simulink model "Control_Pendulo_Simple"  (R2021a)
settings: Solver=ode4  StartTime=0.0  StopTime=100  FixedStep=1e-3  RelTol=1e-3
PreLoadFcn:
  | Control_Pendulo_Simple_Cuentas;
InitFcn:
  | Control_Pendulo_Simple_Cuentas;
values from neighbouring files (symbols this model uses):
  K = acker(sys.A, sys.B, [-3 -3 -2 -2])    [Control_Pendulo_Simple_Cuentas.m]
  Ka = Ka(1:4)    [Control_Pendulo_Simple_Cuentas.m]
  KaDisc = KDisc2(1:4)    [Control_Pendulo_Simple_Cuentas.m]
  Kai = Ka(5)    [Control_Pendulo_Simple_Cuentas.m]
  KaiDisc = KDisc2(5)    [Control_Pendulo_Simple_Cuentas.m]
  KDisc = acker(sysDisc.A, sysDisc.B, exp([-2 -2 -1 -1].*Ts))    [Control_Pendulo_Simple_Cuentas.m]
  L = place((sys.A)',(sys.C)', [-25 -20 -35 -30])'    [Control_Pendulo_Simple_Cuentas.m]
  LDisc = place((sysDisc.A)',(sysDisc.C)', exp([-20 -15 -25 -30].*Ts))'    [Control_Pendulo_Simple_Cuentas.m]
  s = tf('s')    [Control_Pendulo_Simple_Cuentas.m]
  sys = ss(A,B,C,D)    [Control_Pendulo_Simple_Cuentas.m]
  sysDisc = c2d(sys, Ts, 'tustin')    [Control_Pendulo_Simple_Cuentas.m]
  Ts = 0.1    [Control_Pendulo_Simple_Cuentas.m]
  Ts2 = 0.05    [Control_Pendulo_Simple_Cuentas.m]
  Ts_loop = 25/1000    (= 0.025)    [Control_Pendulo_Simple_Cuentas.m]
undefined symbols (not defined in the file or in its folder): C_p_d, C_p_Disc_d, C_p_Disc_n, C_p_n, C_q_d, C_q_Disc_d, C_q_Disc_n, C_q_n, DiscIntNeverNeededParam, X, Y, Z
libraries: sm_lib x84, nesl_utility x42, eeGeneralControl x5
(part 1 of 3)
settings Model: Creator=Acer  LastModifiedBy=Acer

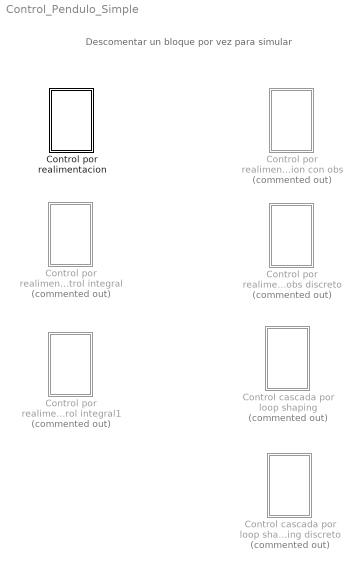
== system Control_Pendulo_Simple ==
  note: Descomentar un bloque por vez para simular
  Control cascada por loop shaping : Subsystem  Commented=on
  Control cascada por loop shaping discreto : Subsystem  Commented=on
  Control por realimentacion : Subsystem
  Control por realimentacion con control integral : Subsystem  Commented=on
  Control por realimentacion con control integral1 : Subsystem  Commented=on
  Control por realimentacion con obs : Subsystem  Commented=on
  Control por realimentacion con obs discreto : Subsystem  Commented=on

== system Control_Pendulo_Simple/Control cascada por loop shaping ==
  note: 2 seg -> Referencia de posición a 5m
      |
      | Notar el error permanente.
  note: Loop shaping de la posición
  Gain : Gain  Gain=-1
  Loop shaping del ángulo : Subsystem
  Pos y Ang : Scope  NumInputPorts=2
  Ref y Pos : Scope  NumInputPorts=2
  Step : Step  Time=2  SampleTime=0
  Sum : Sum  Inputs=|+-
  Transfer Fcn : TransferFcn  Numerator=C_p_n  Denominator=C_p_d
  wires:
  Sum/1 -> Loop shaping del ángulo/1(In1)
  Loop shaping del ángulo/1(Posicion) -> Transfer Fcn/1, Pos y Ang/1, Gain/1
  Loop shaping del ángulo/2(Angulo) -> Pos y Ang/2
  Transfer Fcn/1 -> Sum/2
  Step/1 -> Ref y Pos/1, Sum/1
  Gain/1 -> Ref y Pos/2

== system Control_Pendulo_Simple/Control cascada por loop shaping discreto ==
  note: 2 seg -> Referencia de posición a 5m
      |
      | Notar el error permanente.
  note: Loop shaping de la posición
  Discrete Transfer Fcn : DiscreteTransferFcn  Numerator=C_p_Disc_n  Denominator=C_p_Disc_d  SampleTime=Ts_loop
  Gain : Gain  Gain=-1
  Loop shaping del ángulo : Subsystem
  Pos y Ang : Scope  NumInputPorts=2
  Ref y Pos : Scope  NumInputPorts=2
  Step : Step  Time=2  SampleTime=0
  Sum : Sum  Inputs=|+-
  wires:
  Sum/1 -> Loop shaping del ángulo/1(In1)
  Loop shaping del ángulo/1(Posicion) -> Discrete Transfer Fcn/1, Pos y Ang/1, Gain/1
  Loop shaping del ángulo/2(Angulo) -> Pos y Ang/2
  Discrete Transfer Fcn/1 -> Sum/2
  Step/1 -> Ref y Pos/1, Sum/1
  Gain/1 -> Ref y Pos/2

== system Control_Pendulo_Simple/Control por realimentacion ==
  note: Control por realimentación:
      | 1 seg -> ref de posición a 5m
      | 12 seg -> ref de posición a -5m
      | 25 seg -> disturbio cada 3 segundos
      |
      | Notar el error permanente
  Disturbio : Subsystem
  Gain : Gain  Gain=-K  Multiplication=Matrix(K*u) (u vector)
  Gain1 : Gain  Gain=-1
  Mux : Mux
  Planta : Subsystem  mask{carro_masa=1, barra1_masa=0.25, barra1_long=8}
      mask prompts: carro_masa "Masa del carro"; barra1_masa "Masa primera barra"; barra1_long "Longitud primera barra"
  Pos y Ang : Scope  NumInputPorts=2
  Pos y Ref : Scope  NumInputPorts=2
  Referencia : Subsystem
  Sum : Sum  Inputs=|++
  Sum1 : Sum  Inputs=|++
  wires:
  Mux/1 -> Gain/1
  Planta/1(q) -> Mux/3, Pos y Ang/2  "Angulo"
  Planta/4(v) -> Mux/2  "Velocidad"
  Planta/2(w) -> Mux/4  "Vel Angular"
  Sum/1 -> Planta/1(u)
  Gain/1 -> Sum/2
  Planta/3(p) -> Pos y Ang/1, Pos y Ref/1, Sum1/2  "Posicion"
  Sum1/1 -> Mux/1
  Referencia/1(Posición) -> Gain1/1, Sum1/1
  Disturbio/1(F) -> Sum/1
  Gain1/1 -> Pos y Ref/2

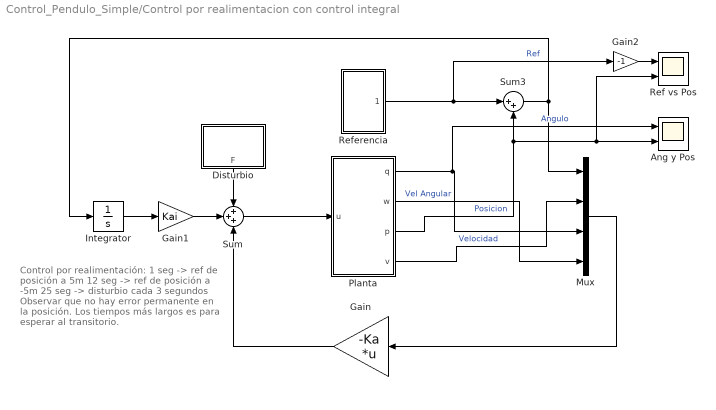
== system Control_Pendulo_Simple/Control por realimentacion con control integral ==
  note: Control por realimentación:
      | 1 seg -> ref de posición a 5m
      | 12 seg -> ref de posición a -5m
      | 25 seg -> disturbio cada 3 segundos
      |
      | Observar que no hay error permanente en la posición. Los tiempos más largos es para esperar al transitorio.
  Ang y Pos : Scope  NumInputPorts=2
  Disturbio : Subsystem
  Gain : Gain  Gain=-Ka  Multiplication=Matrix(K*u) (u vector)
  Gain1 : Gain  Gain=Kai
  Gain2 : Gain  Gain=-1
  Integrator : Integrator
  Mux : Mux
  Planta : Subsystem  mask{carro_masa=1, barra1_masa=0.25, barra1_long=8}
      mask prompts: carro_masa "Masa del carro"; barra1_masa "Masa primera barra"; barra1_long "Longitud primera barra"
  Ref vs Pos : Scope  NumInputPorts=2
  Referencia : Subsystem
  Sum : Sum  Inputs=+++
  Sum3 : Sum  Inputs=|++
  wires:
  Planta/1(q) -> Ang y Pos/1, Mux/3  "Angulo"
  Planta/4(v) -> Mux/2  "Velocidad"
  Gain1/1 -> Sum/2
  Planta/2(w) -> Mux/4  "Vel Angular"
  Sum/1 -> Planta/1(u)
  Mux/1 -> Gain/1
  Gain/1 -> Sum/3
  Sum3/1 -> Integrator/1, Mux/1
  Integrator/1 -> Gain1/1
  Planta/3(p) -> Sum3/2, Ref vs Pos/2, Ang y Pos/2  "Posicion"
  Referencia/1(Posición) -> Gain2/1, Sum3/1  "Ref"
  Disturbio/1(F) -> Sum/1
  Gain2/1 -> Ref vs Pos/1

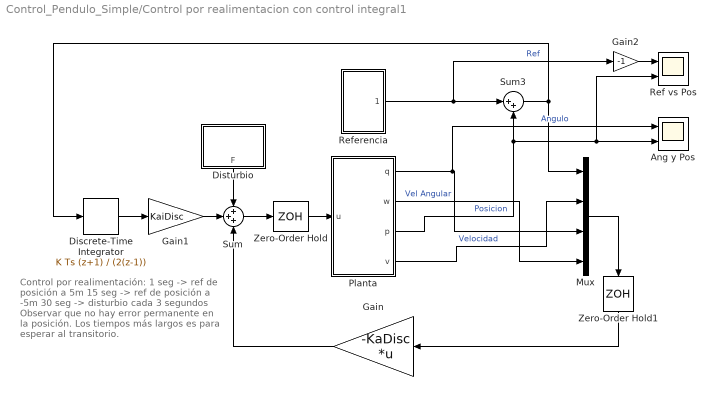
== system Control_Pendulo_Simple/Control por realimentacion con control integral1 ==
  note: Control por realimentación:
      | 1 seg -> ref de posición a 5m
      | 15 seg -> ref de posición a -5m
      | 30 seg -> disturbio cada 3 segundos
      |
      | Observar que no hay error permanente en la posición. Los tiempos más largos es para esperar al transitorio.
  Ang y Pos : Scope  NumInputPorts=2
  Discrete-Time Integrator : DiscreteIntegrator  IntegratorMethod=Integration: Trapezoidal  SampleTime=Ts2  ICPrevOutput=DiscIntNeverNeededParam  ICPrevScaledInput=DiscIntNeverNeededParam
  Disturbio : Subsystem
  Gain : Gain  Gain=-KaDisc  Multiplication=Matrix(K*u) (u vector)
  Gain1 : Gain  Gain=KaiDisc
  Gain2 : Gain  Gain=-1
  Mux : Mux
  Planta : Subsystem  mask{carro_masa=1, barra1_masa=0.25, barra1_long=8}
      mask prompts: carro_masa "Masa del carro"; barra1_masa "Masa primera barra"; barra1_long "Longitud primera barra"
  Ref vs Pos : Scope  NumInputPorts=2
  Referencia : Subsystem
  Sum : Sum  Inputs=+++
  Sum3 : Sum  Inputs=|++
  Zero-Order Hold : ZeroOrderHold  SampleTime=Ts2
  Zero-Order Hold1 : ZeroOrderHold  SampleTime=Ts2
  wires:
  Planta/1(q) -> Ang y Pos/1, Mux/3  "Angulo"
  Planta/4(v) -> Mux/2  "Velocidad"
  Gain1/1 -> Sum/2
  Planta/2(w) -> Mux/4  "Vel Angular"
  Sum/1 -> Zero-Order Hold/1
  Mux/1 -> Zero-Order Hold1/1
  Gain/1 -> Sum/3
  Sum3/1 -> Discrete-Time Integrator/1, Mux/1
  Discrete-Time Integrator/1 -> Gain1/1
  Planta/3(p) -> Sum3/2, Ref vs Pos/2, Ang y Pos/2  "Posicion"
  Referencia/1(Posición) -> Gain2/1, Sum3/1  "Ref"
  Disturbio/1(F) -> Sum/1
  Gain2/1 -> Ref vs Pos/1
  Zero-Order Hold/1 -> Planta/1(u)
  Zero-Order Hold1/1 -> Gain/1

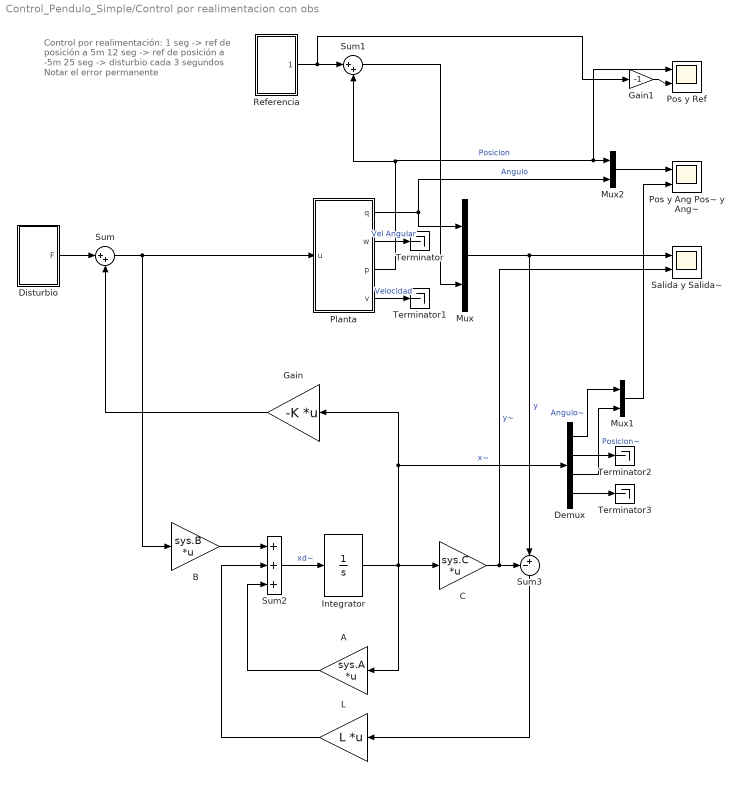
== system Control_Pendulo_Simple/Control por realimentacion con obs ==
  note: Control por realimentación:
      | 1 seg -> ref de posición a 5m
      | 12 seg -> ref de posición a -5m
      | 25 seg -> disturbio cada 3 segundos
      |
      | Notar el error permanente
  A : Gain  Gain=sys.A  Multiplication=Matrix(K*u) (u vector)
  B : Gain  Gain=sys.B  Multiplication=Matrix(K*u) (u vector)
  C : Gain  Gain=sys.C  Multiplication=Matrix(K*u) (u vector)
  Demux : Demux
  Disturbio : Subsystem
  Gain : Gain  Gain=-K  Multiplication=Matrix(K*u) (u vector)
  Gain1 : Gain  Gain=-1
  Integrator : Integrator  InitialCondition=[0 0 0 0]
  L : Gain  Gain=L  Multiplication=Matrix(K*u) (u vector)
  Mux : Mux  Inputs=2
  Mux1 : Mux  Inputs=2
  Mux2 : Mux  Inputs=2
  Planta : Subsystem  mask{carro_masa=1, barra1_masa=0.25, barra1_long=8}
      mask prompts: carro_masa "Masa del carro"; barra1_masa "Masa primera barra"; barra1_long "Longitud primera barra"
  Pos y Ang Pos~ y Ang~ : Scope  NumInputPorts=2
  Pos y Ref : Scope  NumInputPorts=2
  Referencia : Subsystem
  Salida y Salida~ : Scope  NumInputPorts=2
  Sum : Sum  Inputs=|++
  Sum1 : Sum  Inputs=|++
  Sum2 : Sum  Inputs=+++
  Sum3 : Sum  Inputs=-+|
  Terminator{,1..3} (4 alike) : Terminator
  wires:
  Sum/1 -> Planta/1(u), B/1
  Gain/1 -> Sum/2
  Disturbio/1(F) -> Sum/1
  Integrator/1 -> Demux/1, Gain/1, C/1, A/1  "x~"
  Sum2/1 -> Integrator/1  "xd~"
  A/1 -> Sum2/3
  B/1 -> Sum2/1
  Sum3/1 -> L/1
  L/1 -> Sum2/2
  C/1 -> Salida y Salida~/2, Sum3/1  "y~"
  Mux/1 -> Sum3/2, Salida y Salida~/1  "y"
  Sum1/1 -> Mux/2
  Referencia/1(Posición) -> Gain1/1, Sum1/1
  Gain1/1 -> Pos y Ref/2
  Planta/1(q) -> Mux2/2, Mux/1  "Angulo"
  Planta/3(p) -> Mux2/1, Pos y Ref/1, Sum1/2  "Posicion"
  Planta/2(w) -> Terminator/1  "Vel Angular"
  Planta/4(v) -> Terminator1/1  "Velocidad"
  Demux/1 -> Mux1/1  "Angulo~"
  Demux/3 -> Mux1/2  "Posicion~"
  Demux/2 -> Terminator2/1
  Demux/4 -> Terminator3/1
  Mux2/1 -> Pos y Ang Pos~ y Ang~/1
  Mux1/1 -> Pos y Ang Pos~ y Ang~/2

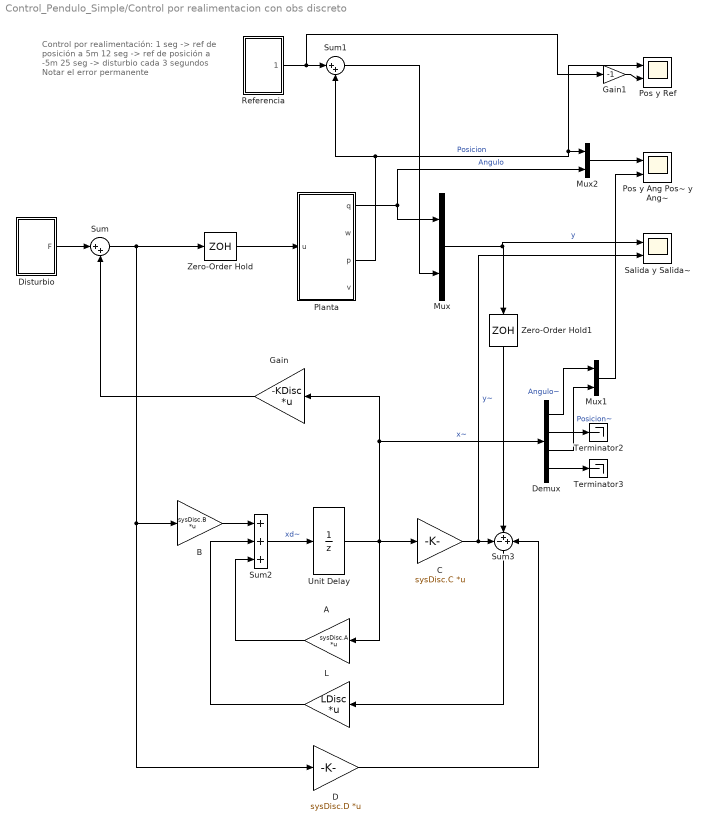
== system Control_Pendulo_Simple/Control por realimentacion con obs discreto ==
  note: Control por realimentación:
      | 1 seg -> ref de posición a 5m
      | 12 seg -> ref de posición a -5m
      | 25 seg -> disturbio cada 3 segundos
      |
      | Notar el error permanente
  A : Gain  Gain=sysDisc.A  Multiplication=Matrix(K*u) (u vector)
  B : Gain  Gain=sysDisc.B  Multiplication=Matrix(K*u) (u vector)
  C : Gain  Gain=sysDisc.C  Multiplication=Matrix(K*u) (u vector)
  D : Gain  Gain=sysDisc.D  Multiplication=Matrix(K*u) (u vector)
  Demux : Demux
  Disturbio : Subsystem
  Gain : Gain  Gain=-KDisc  Multiplication=Matrix(K*u) (u vector)
  Gain1 : Gain  Gain=-1
  L : Gain  Gain=LDisc  Multiplication=Matrix(K*u) (u vector)
  Mux : Mux  Inputs=2
  Mux1 : Mux  Inputs=2
  Mux2 : Mux  Inputs=2
  Planta : Subsystem  mask{carro_masa=1, barra1_masa=0.25, barra1_long=8}
      mask prompts: carro_masa "Masa del carro"; barra1_masa "Masa primera barra"; barra1_long "Longitud primera barra"
  Pos y Ang Pos~ y Ang~ : Scope  NumInputPorts=2
  Pos y Ref : Scope  NumInputPorts=2
  Referencia : Subsystem
  Salida y Salida~ : Scope  NumInputPorts=2
  Sum : Sum  Inputs=|++
  Sum1 : Sum  Inputs=|++
  Sum2 : Sum  Inputs=+++
  Sum3 : Sum  Inputs=-++
  Terminator2 : Terminator
  Terminator3 : Terminator
  Unit Delay : UnitDelay  InitialCondition=[0 0 0 0]  SampleTime=Ts  HasFrameUpgradeWarning=on
  Zero-Order Hold : ZeroOrderHold  SampleTime=Ts
  Zero-Order Hold1 : ZeroOrderHold  SampleTime=Ts
  wires:
  Sum/1 -> Zero-Order Hold/1, B/1, D/1
  Gain/1 -> Sum/2
  Disturbio/1(F) -> Sum/1
  Sum2/1 -> Unit Delay/1  "xd~"
  A/1 -> Sum2/3
  B/1 -> Sum2/1
  Sum3/1 -> L/1
  L/1 -> Sum2/2
  Sum1/1 -> Mux/2
  D/1 -> Sum3/3
  Zero-Order Hold/1 -> Planta/1(u)
  Zero-Order Hold1/1 -> Sum3/2
  Mux1/1 -> Pos y Ang Pos~ y Ang~/2
  Mux2/1 -> Pos y Ang Pos~ y Ang~/1
  Planta/3(p) -> Sum1/2, Mux2/1, Pos y Ref/1  "Posicion"
  Demux/2 -> Terminator2/1
  Demux/3 -> Mux1/2  "Posicion~"
  Planta/1(q) -> Mux2/2, Mux/1  "Angulo"
  Unit Delay/1 -> Demux/1, Gain/1, C/1, A/1  "x~"
  Referencia/1(Posición) -> Gain1/1, Sum1/1
  Mux/1 -> Salida y Salida~/1, Zero-Order Hold1/1  "y"
  Gain1/1 -> Pos y Ref/2
  Demux/1 -> Mux1/1  "Angulo~"
  C/1 -> Salida y Salida~/2, Sum3/1  "y~"
  Demux/4 -> Terminator3/1

== system Control_Pendulo_Simple/Control cascada por loop shaping/Loop shaping del ángulo ==
  In1 : Inport
  Planta : Subsystem  mask{carro_masa=1, barra1_masa=0.25, barra1_long=8}
      mask prompts: carro_masa "Masa del carro"; barra1_masa "Masa primera barra"; barra1_long "Longitud primera barra"
  Sum : Sum  Inputs=|+-
  Transfer Fcn : TransferFcn  Numerator=C_q_n  Denominator=C_q_d
  Posicion : Outport
  Angulo : Outport  Port=2
  wires:
  Planta/2(p) -> Posicion/1  "Posicion"
  Planta/1(q) -> Transfer Fcn/1, Angulo/1  "Angulo"
  In1/1 -> Sum/1
  Sum/1 -> Planta/1(u)
  Transfer Fcn/1 -> Sum/2

== system Control_Pendulo_Simple/Control cascada por loop shaping discreto/Loop shaping del ángulo ==
  In1 : Inport
  Discrete Transfer Fcn : DiscreteTransferFcn  Numerator=C_q_Disc_n  Denominator=C_q_Disc_d  SampleTime=Ts_loop
  Planta : Subsystem  mask{carro_masa=1, barra1_masa=0.25, barra1_long=8}
      mask prompts: carro_masa "Masa del carro"; barra1_masa "Masa primera barra"; barra1_long "Longitud primera barra"
  Sum : Sum  Inputs=|+-
  Zero-Order Hold : ZeroOrderHold  SampleTime=Ts_loop
  Zero-Order Hold1 : ZeroOrderHold  SampleTime=Ts_loop
  Zero-Order Hold2 : ZeroOrderHold  SampleTime=Ts_loop
  Posicion : Outport
  Angulo : Outport  Port=2
  wires:
  Planta/2(p) -> Zero-Order Hold2/1  "Posicion"
  Planta/1(q) -> Zero-Order Hold1/1  "Angulo"
  In1/1 -> Sum/1
  Sum/1 -> Zero-Order Hold/1
  Discrete Transfer Fcn/1 -> Sum/2
  Zero-Order Hold/1 -> Planta/1(u)
  Zero-Order Hold1/1 -> Discrete Transfer Fcn/1, Angulo/1
  Zero-Order Hold2/1 -> Posicion/1

== system Control_Pendulo_Simple/Control por realimentacion/Disturbio ==
  Pulse Generator : DiscretePulseGenerator  PulseType=Time based  Amplitude=500  Period=3  PulseWidth=0.5  PhaseDelay=25
  F : Outport
  wires:
  Pulse Generator/1 -> F/1

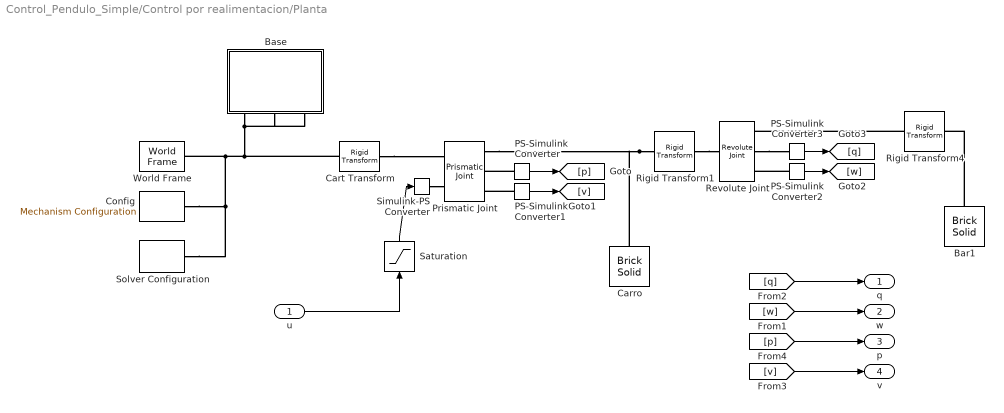
== system Control_Pendulo_Simple/Control por realimentacion/Planta ==
  u : Inport
  Bar1 : sm_lib/Body Elements/Brick Solid  GraphicAmbientColor=[0.15 0.15 0.15 1.0]  BasedOnType=Mass  BrickDimensions=[barra1_long 0.5 0.5]  BrickDimensionUnits=m  CenterOfMass=[0 0 0]  CenterOfMassUnits=m  GraphicDiffuseColor=[1.0 0 0]  Density=1000  DensityUnits=kg/m^3  DoExposeReferenceFrame=off  GraphicEmissiveColor=[0.0 0.0 0.0 1.0]  ExportEntireGeometry=off  SerializedFrames=<Frames><Frame><Id>Frame1</Id><Value><Name>F1</Name><Origin><Source>GeometricFeature</Source><FeatureName>+x surface</FeatureName></Origin><PrimaryAxis><DefinedDirection>+Z</DefinedDirection><Source>ReferenceFrame</Source><SourceDirection>+Z</SourceDirection><FeatureName></FeatureName></PrimaryAxis><SecondaryAxis><DefinedDirection>+X</DefinedDirection><Source>ReferenceFrame</Source><SourceDirection>+X</SourceDirection><FeatureName></FeatureName></SecondaryAxis></Value></Frame></Frames>  MarkerShape=Sphere  MarkerSize=10  GraphicType=FromGeometry  InertiaType=CalculateFromGeometry  Mass=barra1_masa  MassUnits=kg  MomentsOfInertia=[1 1 1]  MomentsOfInertiaUnits=kg*m^2  GraphicOpacity=1.0  ProductsOfInertia=[0 0 0]  ProductsOfInertiaUnits=kg*m^2  GraphicShininess=75  GraphicSpecularColor=[0.5 0.5 0.5 1.0]  GraphicVisPropType=SimpleVisualProperties
  Base : Subsystem
      settings: PortSchema="{\"entries\":[{\"content\":{\"sides\":[{\"content\":{\"connectorIds\":[]},\"type\":\"ConnectorPlacement.EquallySpacedRectSide\",\"uuid\":\"4332d69e-9bfe-4e89-a576-e2f6915cd745\"},{\"content\":{\"connectorIds\":[],\"side\":\"RIGHT\"},\"type\":\"ConnectorPlacement.EquallySpacedRectSide\",\"uuid\":\"1cc8b419-5de1-497b-b007-7cad9f99b098\"},{\"content\":{\"connectorIds\":[],\"side\":\"TOP\"},\"type\":\"ConnectorPlacement.EquallySpacedRectSide\",\"uuid\":\"21186588-641c-464a-a5f8-9ec189ea03bb\"},{\"content\":{\"connectorIds\":[\"RConn1\",\"RConn2\",\"RConn3\"],\"side\":\"BOTTOM\"},\"type\":\"ConnectorPlacement.EquallySpacedRectSide\",\"uuid\":\"3296c54c-d68e-452d-9e4e-a58ba512af2d\"}]},\"type\":\"ConnectorPlacement.EquallySpacedConnector\",\"uuid\":\"cf495630-4c35-4c65-b481-9d90798c8966\"}],\"packageUris\":[\"http://schema.mathworks.com/mf0/Connector/R2020b\"],\"version\":\"1.0\"}"
  Carro : sm_lib/Body Elements/Brick Solid  GraphicAmbientColor=[0.15 0.15 0.15 1.0]  BasedOnType=Mass  BrickDimensions=[0.5 1.5 3]  BrickDimensionUnits=m  CenterOfMass=[0 0 0]  CenterOfMassUnits=m  GraphicDiffuseColor=[1.0 1.0 1.0]  Density=1000  DensityUnits=kg/m^3  DoExposeReferenceFrame=on  GraphicEmissiveColor=[0.0 0.0 0.0 1.0]  ExportEntireGeometry=off  SerializedFrames=<Frames/>  MarkerShape=Sphere  MarkerSize=10  GraphicType=FromGeometry  InertiaType=CalculateFromGeometry  Mass=carro_masa  MassUnits=kg  MomentsOfInertia=[1 1 1]  MomentsOfInertiaUnits=kg*m^2  GraphicOpacity=1.0  ProductsOfInertia=[0 0 0]  ProductsOfInertiaUnits=kg*m^2  GraphicShininess=75  GraphicSpecularColor=[0.5 0.5 0.5 1.0]  GraphicVisPropType=SimpleVisualProperties
  Cart Transform : sm_lib/Frames and Transforms/Rigid Transform  TranslationMethod=StandardAxis  TranslationStandardOffset=0.2  TranslationLengthUnit=m  TranslationStandardAxis=+Z  TranslationCartesianOffset=[0 0 0]  TranslationROffset=0  TranslationROffsetUnits=m  TranslationZOffset=0  TranslationZOffsetUnits=m  TranslationThetaOffset=0  TranslationThetaOffsetUnits=deg  RotationMethod=RotationSequence  RotationAngleUnits=deg  RotationStandardAxis=+Z  RotationAngle=0.0  RotationArbitraryAxis=[0 0 1]  FollAlignAxisA=+X  BaseAlignAxisA=+Y  FollAlignAxisB=+Y  BaseAlignAxisB=+Z  RotationSequenceAxes=FollowerAxes  RotationSequence=XYZ  RotationSequenceAngles=[0 90 0]  RotationSequenceAnglesUnits=deg  RotationMatrix=[1 0 0; 0 1 0; 0 0 1]
  Config : sm_lib/Utilities/Mechanism Configuration  UniformGravity=Constant  GravityVector=[0 0 -9.81]  GravityVectorUnits=m/s^2  GravityUnits=m/s^2  LinearizationDelta=0.001  JointModeTransitionNonlinearIterations=2
  PS-Simulink Converter{,1..3} (4 alike) : nesl_utility/PS-Simulink Converter  PhysicalDomain=network_engine_domain  SubClassName=ps_output  LeftPortType=input  RightPortType=output  PseudoPeriodic=off  Frequencies=[]  Unit=inherit  AffineConversion=off
      settings: SourceProductBaseCode=PW,SS
  Prismatic Joint : sm_lib/Joints/Prismatic Joint  JointMode=Normal  SenseConstraintForce=off  SenseConstraintForceX=off  SenseConstraintForceY=off  SenseConstraintForceZ=off  SenseConstraintTorque=off  SenseConstraintTorqueX=off  SenseConstraintTorqueY=off  SenseConstraintTorqueZ=off  SenseTotalForce=off  SenseTotalForceX=off  SenseTotalForceY=off  SenseTotalForceZ=off  SenseTotalTorque=off  SenseTotalTorqueX=off  SenseTotalTorqueY=off  SenseTotalTorqueZ=off  CompositeWrenchDir=FollowerOnBase  CompositeWrenchFrame=BaseFrame  EquilibriumPosition=0  EquilibriumPositionUnits=m  SpringStiffness=0  SpringStiffnessUnits=N/m  DampingCoefficient=0  DampingCoefficientUnits=N/(m/s)  TorqueActuationMode=InputTorque  MotionActuationMode=ComputedMotion  SensePosition=on  SenseVelocity=on  SenseAcceleration=off  SenseTorqueForce=off  SenseLowerLimitTorqueForce=off  SenseUpperLimitTorqueForce=off  LowerLimitSpecify=off  LowerLimitBound=-10  LowerLimitBoundUnits=m  LowerLimitStiffness=1e6  LowerLimitStiffnessUnits=N/m  LowerLimitDamping=1e3  LowerLimitDampingUnits=N/(m/s)  LowerLimitTransitionRegionWidth=1e-4  LowerLimitTransitionRegionWidthUnits=m  UpperLimitSpecify=off  UpperLimitBound=10  UpperLimitBoundUnits=m  UpperLimitStiffness=1e6  UpperLimitStiffnessUnits=N/m  UpperLimitDamping=1e3  UpperLimitDampingUnits=N/(m/s)  UpperLimitTransitionRegionWidth=1e-4  UpperLimitTransitionRegionWidthUnits=m  PositionTargetSpecify=off  PositionTargetPriority=High  PositionTargetValue=0  PositionTargetValueUnits=m  VelocityTargetSpecify=off  VelocityTargetPriority=High  VelocityTargetValue=0  VelocityTargetValueUnits=m/s
  Revolute Joint : sm_lib/Joints/Revolute Joint  JointMode=Normal  SenseConstraintForce=off  SenseConstraintForceX=off  SenseConstraintForceY=off  SenseConstraintForceZ=off  SenseConstraintTorque=off  SenseConstraintTorqueX=off  SenseConstraintTorqueY=off  SenseConstraintTorqueZ=off  SenseTotalForce=off  SenseTotalForceX=off  SenseTotalForceY=off  SenseTotalForceZ=off  SenseTotalTorque=off  SenseTotalTorqueX=off  SenseTotalTorqueY=off  SenseTotalTorqueZ=off  CompositeWrenchDir=FollowerOnBase  CompositeWrenchFrame=BaseFrame  EquilibriumPosition=0  EquilibriumPositionUnits=deg  SpringStiffness=0  SpringStiffnessUnits=N*m/deg  DampingCoefficient=0  DampingCoefficientUnits=N*m/(deg/s)  TorqueActuationMode=NoTorque  MotionActuationMode=ComputedMotion  SensePosition=on  SenseVelocity=on  SenseAcceleration=off  SenseTorqueForce=off  SenseLowerLimitTorqueForce=off  SenseUpperLimitTorqueForce=off  LowerLimitSpecify=off  LowerLimitBound=-90  LowerLimitBoundUnits=deg  LowerLimitStiffness=1e4  LowerLimitStiffnessUnits=N*m/deg  LowerLimitDamping=10  LowerLimitDampingUnits=N*m/(deg/s)  LowerLimitTransitionRegionWidth=0.1  LowerLimitTransitionRegionWidthUnits=deg  UpperLimitSpecify=off  UpperLimitBound=90  UpperLimitBoundUnits=deg  UpperLimitStiffness=1e4  UpperLimitStiffnessUnits=N*m/deg  UpperLimitDamping=10  UpperLimitDampingUnits=N*m/(deg/s)  UpperLimitTransitionRegionWidth=0.1  UpperLimitTransitionRegionWidthUnits=deg  PositionTargetSpecify=off  PositionTargetPriority=Low  PositionTargetValue=0.001  PositionTargetValueUnits=deg  VelocityTargetSpecify=off  VelocityTargetPriority=High  VelocityTargetValue=0  VelocityTargetValueUnits=deg/s
  Rigid Transform1 : sm_lib/Frames and Transforms/Rigid Transform  TranslationMethod=StandardAxis  TranslationStandardOffset=0  TranslationLengthUnit=m  TranslationStandardAxis=+X  TranslationCartesianOffset=[0 0 0]  TranslationROffset=0  TranslationROffsetUnits=m  TranslationZOffset=0  TranslationZOffsetUnits=m  TranslationThetaOffset=0  TranslationThetaOffsetUnits=deg  RotationMethod=RotationSequence  RotationAngleUnits=deg  RotationStandardAxis=+Z  RotationAngle=0.0  RotationArbitraryAxis=[0 0 1]  FollAlignAxisA=+X  BaseAlignAxisA=+Y  FollAlignAxisB=+Y  BaseAlignAxisB=+Z  RotationSequenceAxes=FollowerAxes  RotationSequence=XYZ  RotationSequenceAngles=[90 0 0.1]  RotationSequenceAnglesUnits=deg  RotationMatrix=[1 0 0; 0 1 0; 0 0 1]
  Rigid Transform4 : sm_lib/Frames and Transforms/Rigid Transform  TranslationMethod=StandardAxis  TranslationStandardOffset=0  TranslationLengthUnit=m  TranslationStandardAxis=+Z  TranslationCartesianOffset=[0 0 0]  TranslationROffset=0  TranslationROffsetUnits=m  TranslationZOffset=0  TranslationZOffsetUnits=m  TranslationThetaOffset=0  TranslationThetaOffsetUnits=deg  RotationMethod=RotationSequence  RotationAngleUnits=deg  RotationStandardAxis=+Z  RotationAngle=0.0  RotationArbitraryAxis=[0 0 1]  FollAlignAxisA=+X  BaseAlignAxisA=+Y  FollAlignAxisB=+Y  BaseAlignAxisB=+Z  RotationSequenceAxes=FollowerAxes  RotationSequence=XYZ  RotationSequenceAngles=[0 0 0]  RotationSequenceAnglesUnits=deg  RotationMatrix=[1 0 0; 0 1 0; 0 0 1]
  Saturation : Saturate  UpperLimit=1000  LowerLimit=-1000
  Simulink-PS Converter : nesl_utility/Simulink-PS Converter  PhysicalDomain=network_engine_domain  SubClassName=ps_input  LeftPortType=input  RightPortType=output  PseudoPeriodic=off  Frequencies=[]  NoiseDistribution=none  NoiseParameters=[]  Unit=1  AffineConversion=off  FilteringAndDerivatives=provide  SimscapeFilterOrder=1  InputFilterTimeConstant=0.001  UdotUserProvided=0
      settings: SourceProductBaseCode=PW,SS
  Solver Configuration : nesl_utility/Solver Configuration  PhysicalDomain=network_engine_domain  SubClassName=solver  LeftPortType=input  RightPortType=generic  Tones=[]  Harmonics=[]  SimulateNoise=off  Profile=off  UseLocalSampling=off  EnableSwitchedLinearOptims=on  FrequencyDomain=off  UseCCode=off  RelTol=0.001  AbsTol=1e-06  MinStep=1e-09  ToWorkspace=off  RevertToSquareIcSolve=off  NumHomotopyIterations=100  PhasorMode=off  PhasorModeNumHarmonics=1  DoDC=off  ResidualTolerance=1e-09  UseLocalSolver=off  LocalSolverChoice=NE_BACKWARD_EULER_ADVANCER  LocalSolverSampleTime=0.001  DoFixedCost=off  MaxNonlinIter=3  MaxModeIter=2  ComputeImpulses=off  ImpulseIterations=2  LinearAlgebra=auto  EquationFormulation=NE_TIME_EF  DelaysMemoryBudget=1024  AutomaticFiltering=on  FilteringTimeConstant=0.001  PartitionStorageMethod=AS_NEEDED  PartitionMemoryBudget=1024  PartitionMethod=ROBUST
      settings: SourceProductBaseCode=PW,SS
  World Frame : sm_lib/Frames and Transforms/World Frame
  q : Outport
  w : Outport  Port=2
  p : Outport  Port=3
  v : Outport  Port=4
  wires:
  u/1 -> Saturation/1
  PS-Simulink Converter/1 -> [p]
  PS-Simulink Converter3/1 -> [q]
  [q] -> q/1
  [p] -> p/1
  PS-Simulink Converter1/1 -> [v]
  PS-Simulink Converter2/1 -> [w]
  [w] -> w/1
  [v] -> v/1
  Saturation/1 -> Simulink-PS Converter/1
  connections:
  PS-Simulink Converter1/LConn1 -- Prismatic Joint/RConn3
  Bar1/LConn1 -- Rigid Transform4/RConn1
  Rigid Transform4/LConn1 -- Revolute Joint/RConn1
  Config/RConn1 -- Solver Configuration/RConn1 -- Cart Transform/LConn1 -- Base/RConn3 -- Base/RConn2 -- Base/RConn1 -- World Frame/RConn1
  Cart Transform/RConn1 -- Prismatic Joint/LConn1
  PS-Simulink Converter/LConn1 -- Prismatic Joint/RConn2
  Simulink-PS Converter/RConn1 -- Prismatic Joint/LConn2
  PS-Simulink Converter2/LConn1 -- Revolute Joint/RConn3
  Rigid Transform1/RConn1 -- Revolute Joint/LConn1
  Revolute Joint/RConn2 -- PS-Simulink Converter3/LConn1
  Rigid Transform1/LConn1 -- Prismatic Joint/RConn1 -- Carro/RConn1

== system Control_Pendulo_Simple/Control por realimentacion/Referencia ==
  note: Pre-filtro para no irse mucho del punto de linealización
  Low-Pass Filter (Discrete or Continuous) : eeGeneralControl/Low-Pass Filter (Discrete or Continuous)  K=1  T=1  B=inf  A=-inf  init_option=Inherited from block input  x0=0  Ts=-1
  Step1 : Step  After=2  SampleTime=0
  Step2 : Step  Time=12  After=-4  SampleTime=0
  Sum2 : Sum  Inputs=|++
  Posición : Outport
  wires:
  Step2/1 -> Sum2/2
  Sum2/1 -> Low-Pass Filter (Discrete or Continuous)/1
  Low-Pass Filter (Discrete or Continuous)/1 -> Posición/1
  Step1/1 -> Sum2/1

== system Control_Pendulo_Simple/Control por realimentacion con control integral/Disturbio ==
  Pulse Generator : DiscretePulseGenerator  PulseType=Time based  Amplitude=500  Period=5  PulseWidth=0.5  PhaseDelay=25
  F : Outport
  wires:
  Pulse Generator/1 -> F/1

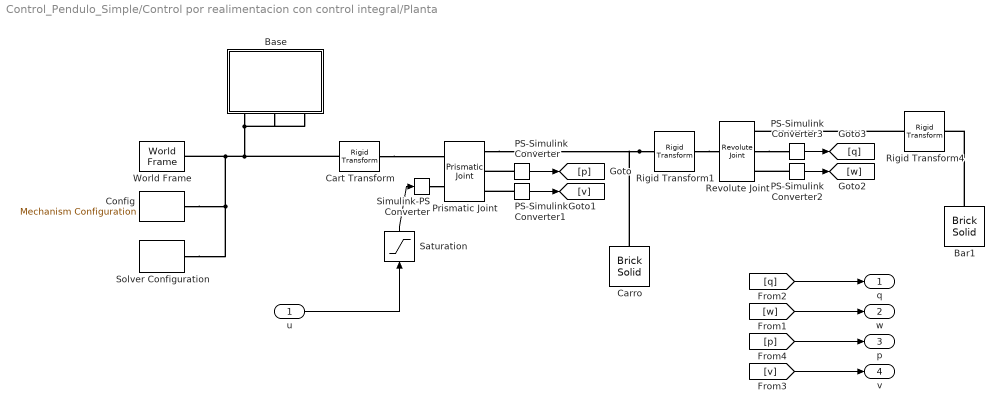
== system Control_Pendulo_Simple/Control por realimentacion con control integral/Planta ==
  u : Inport
  Bar1 : sm_lib/Body Elements/Brick Solid  GraphicAmbientColor=[0.15 0.15 0.15 1.0]  BasedOnType=Mass  BrickDimensions=[barra1_long 0.5 0.5]  BrickDimensionUnits=m  CenterOfMass=[0 0 0]  CenterOfMassUnits=m  GraphicDiffuseColor=[1.0 0 0]  Density=1000  DensityUnits=kg/m^3  DoExposeReferenceFrame=off  GraphicEmissiveColor=[0.0 0.0 0.0 1.0]  ExportEntireGeometry=off  SerializedFrames=<Frames><Frame><Id>Frame1</Id><Value><Name>F1</Name><Origin><Source>GeometricFeature</Source><FeatureName>+x surface</FeatureName></Origin><PrimaryAxis><DefinedDirection>+Z</DefinedDirection><Source>ReferenceFrame</Source><SourceDirection>+Z</SourceDirection><FeatureName></FeatureName></PrimaryAxis><SecondaryAxis><DefinedDirection>+X</DefinedDirection><Source>ReferenceFrame</Source><SourceDirection>+X</SourceDirection><FeatureName></FeatureName></SecondaryAxis></Value></Frame></Frames>  MarkerShape=Sphere  MarkerSize=10  GraphicType=FromGeometry  InertiaType=CalculateFromGeometry  Mass=barra1_masa  MassUnits=kg  MomentsOfInertia=[1 1 1]  MomentsOfInertiaUnits=kg*m^2  GraphicOpacity=1.0  ProductsOfInertia=[0 0 0]  ProductsOfInertiaUnits=kg*m^2  GraphicShininess=75  GraphicSpecularColor=[0.5 0.5 0.5 1.0]  GraphicVisPropType=SimpleVisualProperties
  Base : Subsystem
      settings: PortSchema="{\"entries\":[{\"content\":{\"sides\":[{\"content\":{\"connectorIds\":[]},\"type\":\"ConnectorPlacement.EquallySpacedRectSide\",\"uuid\":\"4332d69e-9bfe-4e89-a576-e2f6915cd745\"},{\"content\":{\"connectorIds\":[],\"side\":\"RIGHT\"},\"type\":\"ConnectorPlacement.EquallySpacedRectSide\",\"uuid\":\"1cc8b419-5de1-497b-b007-7cad9f99b098\"},{\"content\":{\"connectorIds\":[],\"side\":\"TOP\"},\"type\":\"ConnectorPlacement.EquallySpacedRectSide\",\"uuid\":\"21186588-641c-464a-a5f8-9ec189ea03bb\"},{\"content\":{\"connectorIds\":[\"RConn1\",\"RConn2\",\"RConn3\"],\"side\":\"BOTTOM\"},\"type\":\"ConnectorPlacement.EquallySpacedRectSide\",\"uuid\":\"3296c54c-d68e-452d-9e4e-a58ba512af2d\"}]},\"type\":\"ConnectorPlacement.EquallySpacedConnector\",\"uuid\":\"cf495630-4c35-4c65-b481-9d90798c8966\"}],\"packageUris\":[\"http://schema.mathworks.com/mf0/Connector/R2020b\"],\"version\":\"1.0\"}"
  Carro : sm_lib/Body Elements/Brick Solid  GraphicAmbientColor=[0.15 0.15 0.15 1.0]  BasedOnType=Mass  BrickDimensions=[0.5 1.5 3]  BrickDimensionUnits=m  CenterOfMass=[0 0 0]  CenterOfMassUnits=m  GraphicDiffuseColor=[1.0 1.0 1.0]  Density=1000  DensityUnits=kg/m^3  DoExposeReferenceFrame=on  GraphicEmissiveColor=[0.0 0.0 0.0 1.0]  ExportEntireGeometry=off  SerializedFrames=<Frames/>  MarkerShape=Sphere  MarkerSize=10  GraphicType=FromGeometry  InertiaType=CalculateFromGeometry  Mass=carro_masa  MassUnits=kg  MomentsOfInertia=[1 1 1]  MomentsOfInertiaUnits=kg*m^2  GraphicOpacity=1.0  ProductsOfInertia=[0 0 0]  ProductsOfInertiaUnits=kg*m^2  GraphicShininess=75  GraphicSpecularColor=[0.5 0.5 0.5 1.0]  GraphicVisPropType=SimpleVisualProperties
  Cart Transform : sm_lib/Frames and Transforms/Rigid Transform  TranslationMethod=StandardAxis  TranslationStandardOffset=0.2  TranslationLengthUnit=m  TranslationStandardAxis=+Z  TranslationCartesianOffset=[0 0 0]  TranslationROffset=0  TranslationROffsetUnits=m  TranslationZOffset=0  TranslationZOffsetUnits=m  TranslationThetaOffset=0  TranslationThetaOffsetUnits=deg  RotationMethod=RotationSequence  RotationAngleUnits=deg  RotationStandardAxis=+Z  RotationAngle=0.0  RotationArbitraryAxis=[0 0 1]  FollAlignAxisA=+X  BaseAlignAxisA=+Y  FollAlignAxisB=+Y  BaseAlignAxisB=+Z  RotationSequenceAxes=FollowerAxes  RotationSequence=XYZ  RotationSequenceAngles=[0 90 0]  RotationSequenceAnglesUnits=deg  RotationMatrix=[1 0 0; 0 1 0; 0 0 1]
  Config : sm_lib/Utilities/Mechanism Configuration  UniformGravity=Constant  GravityVector=[0 0 -9.81]  GravityVectorUnits=m/s^2  GravityUnits=m/s^2  LinearizationDelta=0.001  JointModeTransitionNonlinearIterations=2
  PS-Simulink Converter{,1..3} (4 alike) : nesl_utility/PS-Simulink Converter  PhysicalDomain=network_engine_domain  SubClassName=ps_output  LeftPortType=input  RightPortType=output  PseudoPeriodic=off  Frequencies=[]  Unit=inherit  AffineConversion=off
      settings: SourceProductBaseCode=PW,SS
  Prismatic Joint : sm_lib/Joints/Prismatic Joint  JointMode=Normal  SenseConstraintForce=off  SenseConstraintForceX=off  SenseConstraintForceY=off  SenseConstraintForceZ=off  SenseConstraintTorque=off  SenseConstraintTorqueX=off  SenseConstraintTorqueY=off  SenseConstraintTorqueZ=off  SenseTotalForce=off  SenseTotalForceX=off  SenseTotalForceY=off  SenseTotalForceZ=off  SenseTotalTorque=off  SenseTotalTorqueX=off  SenseTotalTorqueY=off  SenseTotalTorqueZ=off  CompositeWrenchDir=FollowerOnBase  CompositeWrenchFrame=BaseFrame  EquilibriumPosition=0  EquilibriumPositionUnits=m  SpringStiffness=0  SpringStiffnessUnits=N/m  DampingCoefficient=0  DampingCoefficientUnits=N/(m/s)  TorqueActuationMode=InputTorque  MotionActuationMode=ComputedMotion  SensePosition=on  SenseVelocity=on  SenseAcceleration=off  SenseTorqueForce=off  SenseLowerLimitTorqueForce=off  SenseUpperLimitTorqueForce=off  LowerLimitSpecify=off  LowerLimitBound=-10  LowerLimitBoundUnits=m  LowerLimitStiffness=1e6  LowerLimitStiffnessUnits=N/m  LowerLimitDamping=1e3  LowerLimitDampingUnits=N/(m/s)  LowerLimitTransitionRegionWidth=1e-4  LowerLimitTransitionRegionWidthUnits=m  UpperLimitSpecify=off  UpperLimitBound=10  UpperLimitBoundUnits=m  UpperLimitStiffness=1e6  UpperLimitStiffnessUnits=N/m  UpperLimitDamping=1e3  UpperLimitDampingUnits=N/(m/s)  UpperLimitTransitionRegionWidth=1e-4  UpperLimitTransitionRegionWidthUnits=m  PositionTargetSpecify=off  PositionTargetPriority=High  PositionTargetValue=0  PositionTargetValueUnits=m  VelocityTargetSpecify=off  VelocityTargetPriority=High  VelocityTargetValue=0  VelocityTargetValueUnits=m/s
  Revolute Joint : sm_lib/Joints/Revolute Joint  JointMode=Normal  SenseConstraintForce=off  SenseConstraintForceX=off  SenseConstraintForceY=off  SenseConstraintForceZ=off  SenseConstraintTorque=off  SenseConstraintTorqueX=off  SenseConstraintTorqueY=off  SenseConstraintTorqueZ=off  SenseTotalForce=off  SenseTotalForceX=off  SenseTotalForceY=off  SenseTotalForceZ=off  SenseTotalTorque=off  SenseTotalTorqueX=off  SenseTotalTorqueY=off  SenseTotalTorqueZ=off  CompositeWrenchDir=FollowerOnBase  CompositeWrenchFrame=BaseFrame  EquilibriumPosition=0  EquilibriumPositionUnits=deg  SpringStiffness=0  SpringStiffnessUnits=N*m/deg  DampingCoefficient=0  DampingCoefficientUnits=N*m/(deg/s)  TorqueActuationMode=NoTorque  MotionActuationMode=ComputedMotion  SensePosition=on  SenseVelocity=on  SenseAcceleration=off  SenseTorqueForce=off  SenseLowerLimitTorqueForce=off  SenseUpperLimitTorqueForce=off  LowerLimitSpecify=off  LowerLimitBound=-90  LowerLimitBoundUnits=deg  LowerLimitStiffness=1e4  LowerLimitStiffnessUnits=N*m/deg  LowerLimitDamping=10  LowerLimitDampingUnits=N*m/(deg/s)  LowerLimitTransitionRegionWidth=0.1  LowerLimitTransitionRegionWidthUnits=deg  UpperLimitSpecify=off  UpperLimitBound=90  UpperLimitBoundUnits=deg  UpperLimitStiffness=1e4  UpperLimitStiffnessUnits=N*m/deg  UpperLimitDamping=10  UpperLimitDampingUnits=N*m/(deg/s)  UpperLimitTransitionRegionWidth=0.1  UpperLimitTransitionRegionWidthUnits=deg  PositionTargetSpecify=off  PositionTargetPriority=Low  PositionTargetValue=0.001  PositionTargetValueUnits=deg  VelocityTargetSpecify=off  VelocityTargetPriority=High  VelocityTargetValue=0  VelocityTargetValueUnits=deg/s
  Rigid Transform1 : sm_lib/Frames and Transforms/Rigid Transform  TranslationMethod=StandardAxis  TranslationStandardOffset=0  TranslationLengthUnit=m  TranslationStandardAxis=+X  TranslationCartesianOffset=[0 0 0]  TranslationROffset=0  TranslationROffsetUnits=m  TranslationZOffset=0  TranslationZOffsetUnits=m  TranslationThetaOffset=0  TranslationThetaOffsetUnits=deg  RotationMethod=RotationSequence  RotationAngleUnits=deg  RotationStandardAxis=+Z  RotationAngle=0.0  RotationArbitraryAxis=[0 0 1]  FollAlignAxisA=+X  BaseAlignAxisA=+Y  FollAlignAxisB=+Y  BaseAlignAxisB=+Z  RotationSequenceAxes=FollowerAxes  RotationSequence=XYZ  RotationSequenceAngles=[90 0 0.1]  RotationSequenceAnglesUnits=deg  RotationMatrix=[1 0 0; 0 1 0; 0 0 1]
  Rigid Transform4 : sm_lib/Frames and Transforms/Rigid Transform  TranslationMethod=StandardAxis  TranslationStandardOffset=0  TranslationLengthUnit=m  TranslationStandardAxis=+Z  TranslationCartesianOffset=[0 0 0]  TranslationROffset=0  TranslationROffsetUnits=m  TranslationZOffset=0  TranslationZOffsetUnits=m  TranslationThetaOffset=0  TranslationThetaOffsetUnits=deg  RotationMethod=RotationSequence  RotationAngleUnits=deg  RotationStandardAxis=+Z  RotationAngle=0.0  RotationArbitraryAxis=[0 0 1]  FollAlignAxisA=+X  BaseAlignAxisA=+Y  FollAlignAxisB=+Y  BaseAlignAxisB=+Z  RotationSequenceAxes=FollowerAxes  RotationSequence=XYZ  RotationSequenceAngles=[0 0 0]  RotationSequenceAnglesUnits=deg  RotationMatrix=[1 0 0; 0 1 0; 0 0 1]
  Saturation : Saturate  UpperLimit=1000  LowerLimit=-1000
  Simulink-PS Converter : nesl_utility/Simulink-PS Converter  PhysicalDomain=network_engine_domain  SubClassName=ps_input  LeftPortType=input  RightPortType=output  PseudoPeriodic=off  Frequencies=[]  NoiseDistribution=none  NoiseParameters=[]  Unit=1  AffineConversion=off  FilteringAndDerivatives=provide  SimscapeFilterOrder=1  InputFilterTimeConstant=0.001  UdotUserProvided=0
      settings: SourceProductBaseCode=PW,SS
  Solver Configuration : nesl_utility/Solver Configuration  PhysicalDomain=network_engine_domain  SubClassName=solver  LeftPortType=input  RightPortType=generic  Tones=[]  Harmonics=[]  SimulateNoise=off  Profile=off  UseLocalSampling=off  EnableSwitchedLinearOptims=on  FrequencyDomain=off  UseCCode=off  RelTol=0.001  AbsTol=1e-06  MinStep=1e-09  ToWorkspace=off  RevertToSquareIcSolve=off  NumHomotopyIterations=100  PhasorMode=off  PhasorModeNumHarmonics=1  DoDC=off  ResidualTolerance=1e-09  UseLocalSolver=off  LocalSolverChoice=NE_BACKWARD_EULER_ADVANCER  LocalSolverSampleTime=0.001  DoFixedCost=off  MaxNonlinIter=3  MaxModeIter=2  ComputeImpulses=off  ImpulseIterations=2  LinearAlgebra=auto  EquationFormulation=NE_TIME_EF  DelaysMemoryBudget=1024  AutomaticFiltering=on  FilteringTimeConstant=0.001  PartitionStorageMethod=AS_NEEDED  PartitionMemoryBudget=1024  PartitionMethod=ROBUST
      settings: SourceProductBaseCode=PW,SS
  World Frame : sm_lib/Frames and Transforms/World Frame
  q : Outport
  w : Outport  Port=2
  p : Outport  Port=3
  v : Outport  Port=4
  wires:
  u/1 -> Saturation/1
  PS-Simulink Converter/1 -> [p]
  PS-Simulink Converter3/1 -> [q]
  [q] -> q/1
  [p] -> p/1
  PS-Simulink Converter1/1 -> [v]
  PS-Simulink Converter2/1 -> [w]
  [w] -> w/1
  [v] -> v/1
  Saturation/1 -> Simulink-PS Converter/1
  connections:
  PS-Simulink Converter1/LConn1 -- Prismatic Joint/RConn3
  Bar1/LConn1 -- Rigid Transform4/RConn1
  Rigid Transform4/LConn1 -- Revolute Joint/RConn1
  Config/RConn1 -- Solver Configuration/RConn1 -- Cart Transform/LConn1 -- Base/RConn3 -- Base/RConn2 -- Base/RConn1 -- World Frame/RConn1
  Cart Transform/RConn1 -- Prismatic Joint/LConn1
  PS-Simulink Converter/LConn1 -- Prismatic Joint/RConn2
  Simulink-PS Converter/RConn1 -- Prismatic Joint/LConn2
  PS-Simulink Converter2/LConn1 -- Revolute Joint/RConn3
  Rigid Transform1/RConn1 -- Revolute Joint/LConn1
  Revolute Joint/RConn2 -- PS-Simulink Converter3/LConn1
  Rigid Transform1/LConn1 -- Prismatic Joint/RConn1 -- Carro/RConn1

== system Control_Pendulo_Simple/Control por realimentacion con control integral/Referencia ==
  note: Pre-filtro para no irse mucho del punto de linealización
  Low-Pass Filter (Discrete or Continuous) : eeGeneralControl/Low-Pass Filter (Discrete or Continuous)  K=1  T=1  B=inf  A=-inf  init_option=Inherited from block input  x0=0  Ts=-1
  Step1 : Step  After=2  SampleTime=0
  Step2 : Step  Time=12  After=-4  SampleTime=0
  Sum2 : Sum  Inputs=|++
  Posición : Outport
  wires:
  Step2/1 -> Sum2/2
  Sum2/1 -> Low-Pass Filter (Discrete or Continuous)/1
  Low-Pass Filter (Discrete or Continuous)/1 -> Posición/1
  Step1/1 -> Sum2/1

== system Control_Pendulo_Simple/Control por realimentacion con control integral1/Disturbio ==
  Pulse Generator : DiscretePulseGenerator  PulseType=Time based  Amplitude=50  Period=5  PulseWidth=0.5  PhaseDelay=30
  F : Outport
  wires:
  Pulse Generator/1 -> F/1
